simulink subsystem "PvtSubSys_LATC"  (R2020b)
settings: Solver=VariableStepAuto  StartTime=0.0  StopTime=10.0  RelTol=1e-3
undefined symbols (not defined in the file or in its folder): LCS_PLAN_PreViewIdxNum, LCS_PLAN_PreViewIdxSW_b, P_Global_CharSpd_ms, P_Global_SteeringAngleRatio, P_Global_WheelBase_m, P_LCS_DetNoOverRide_DrvTrq_TH, P_LCS_DetOverRide_DrvTrq_TH, P_LCS_ESS_AngleSlope_Limit, P_LCS_ESS_LogicTest_Enable, P_LCS_ESS_NotActiveFlgDelayTime, P_LCS_ESS_NotActiveFlgDelayTimeSW, P_LCS_ESS_SteerAngleErr, P_LCS_ESS_SteerAngleFilterTime, P_LCS_ESS_TarAngleFilterTime, P_LCS_ESSAngleSW, P_LCS_ESSOverrideTime1, P_LCS_ESSOverrideTime2, P_LCS_ESSOverrideTime3, P_LCS_ESSOverrideValue1, P_LCS_ESSOverrideValue2, P_LCS_IN_Offset_Test_SW, P_LCS_IN_Offset_Test_Value, P_LCS_LATC_AngleFilterTime_s, P_LCS_LATC_CurOffsetCurve_TabX_m, P_LCS_LATC_CurOffsetCurveFliterTime_Tab_s, P_LCS_LATC_CurOffsetVehicleSpdLimitValue_degs, P_LCS_LATC_DeltaEps_Tab_s, P_LCS_LATC_DxOffset_Sw, P_LCS_LATC_ELKAngleSlope_ratio, P_LCS_LATC_ELKMaxLatAcc_ms2, P_LCS_LATC_ESSA0Dis_TabX_m, P_LCS_LATC_ESSAddAngleSlope_Tab_degs, P_LCS_LATC_ESSAESAngleSlope_Tab_degs, P_LCS_LATC_ESSAngleSlope_ratio, P_LCS_LATC_ESSMaxLatAcc_ms2, P_LCS_LATC_LCAngleSlope_ratio, P_LCS_LATC_LCAngleSlope_Tab_degs, P_LCS_LATC_LCCancleMaxLatAcc_ms2, P_LCS_LATC_LCEcoAngleSlope_ratio, P_LCS_LATC_LCEcoAngleSlope_Tab_degs, P_LCS_LATC_LCEcoMaxLatAcc_ms2, P_LCS_LATC_LCKAngleSlope_ratio, P_LCS_LATC_LCKAngleSlope_Tab_degs, P_LCS_LATC_LCKIEAngleSlope_ratio, P_LCS_LATC_LCKIEAngleSlope_Tab_degs, P_LCS_LATC_LCKIEMaxLatAcc_ms2, P_LCS_LATC_LCKMaxLatAcc_ms2, P_LCS_LATC_LCNormalAngleSlope_ratio, P_LCS_LATC_LCNormalAngleSlope_Tab_degs, P_LCS_LATC_LCNormalMaxLatAcc_ms2, P_LCS_LATC_LCSportAngleSlope_ratio, P_LCS_LATC_LCSportAngleSlope_Tab_degs, P_LCS_LATC_LCSportMaxLatAcc_ms2, P_LCS_LATC_LKAAngleSlope_ratio, P_LCS_LATC_LKAAngleSlope_Tab_degs, P_LCS_LATC_LKAMaxLatAcc_ms2, P_LCS_LATC_MatrixQ1_st, P_LCS_LATC_MatrixQ3_st, P_LCS_LATC_MatrixR_st, P_LCS_LATC_MPCDeltaT_s ... (+70)
libraries: simulink x34
(part 1 of 5)
settings Model: Creator=GW00184765  LastModifiedBy=GW00201118

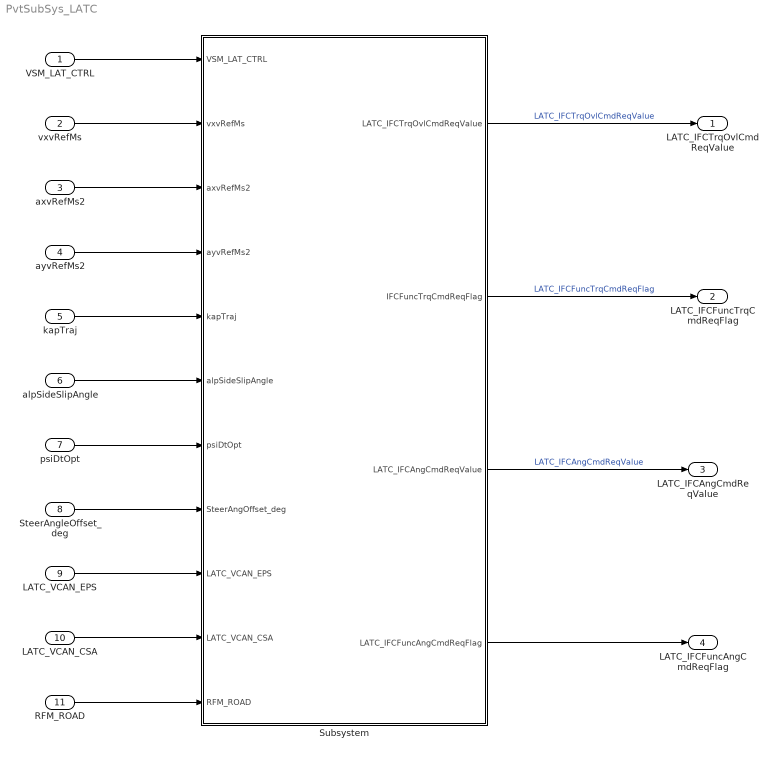
== system PvtSubSys_LATC ==
  VSM_LAT_CTRL : Inport  OutDataTypeStr=Bus: VSM_LAT_CTRL_BUS  PortDimensions=1  BusOutputAsStruct=on
  vxvRefMs : Inport  Port=2  OutDataTypeStr=single  PortDimensions=1  BusOutputAsStruct=on
  axvRefMs2 : Inport  Port=3  OutDataTypeStr=single  PortDimensions=1  BusOutputAsStruct=on
  ayvRefMs2 : Inport  Port=4  OutDataTypeStr=single  PortDimensions=1  BusOutputAsStruct=on
  kapTraj : Inport  Port=5  OutDataTypeStr=single  PortDimensions=1  BusOutputAsStruct=on
  alpSideSlipAngle : Inport  Port=6  OutDataTypeStr=single  PortDimensions=1  BusOutputAsStruct=on
  psiDtOpt : Inport  Port=7  OutDataTypeStr=single  PortDimensions=1  BusOutputAsStruct=on
  SteerAngleOffset_deg : Inport  Port=8  OutDataTypeStr=single  PortDimensions=1  BusOutputAsStruct=on
  LATC_VCAN_EPS : Inport  Port=9  OutDataTypeStr=Bus: VCAN_EPS_MSG_BUS  PortDimensions=1  BusOutputAsStruct=on
  LATC_VCAN_CSA : Inport  Port=10  OutDataTypeStr=Bus: VCAN_CSA_MSG_BUS  PortDimensions=1  BusOutputAsStruct=on
  RFM_ROAD : Inport  Port=11  OutDataTypeStr=Bus: RFM_ROAD_BUS  PortDimensions=1  BusOutputAsStruct=on
  Subsystem : Subsystem
  LATC_IFCTrqOvlCmdReqValue : Outport  OutDataTypeStr=single  PortDimensions=1  BusOutputAsStruct=on
  LATC_IFCFuncTrqCmdReqFlag : Outport  Port=2  OutDataTypeStr=uint8  PortDimensions=1  BusOutputAsStruct=on
  LATC_IFCAngCmdReqValue : Outport  Port=3  OutDataTypeStr=single  PortDimensions=1  BusOutputAsStruct=on
  LATC_IFCFuncAngCmdReqFlag : Outport  Port=4  OutDataTypeStr=uint8  PortDimensions=1  BusOutputAsStruct=on
  wires:
  Subsystem/1(LATC_IFCTrqOvlCmdReqValue) -> LATC_IFCTrqOvlCmdReqValue/1  "LATC_IFCTrqOvlCmdReqValue"
  RFM_ROAD/1 -> Subsystem/11(RFM_ROAD)
  kapTraj/1 -> Subsystem/5(kapTraj)
  vxvRefMs/1 -> Subsystem/2(vxvRefMs)
  alpSideSlipAngle/1 -> Subsystem/6(alpSideSlipAngle)
  ayvRefMs2/1 -> Subsystem/4(ayvRefMs2)
  LATC_VCAN_EPS/1 -> Subsystem/9(LATC_VCAN_EPS)
  Subsystem/2(IFCFuncTrqCmdReqFlag) -> LATC_IFCFuncTrqCmdReqFlag/1  "LATC_IFCFuncTrqCmdReqFlag"
  psiDtOpt/1 -> Subsystem/7(psiDtOpt)
  SteerAngleOffset_deg/1 -> Subsystem/8(SteerAngOffset_deg)
  VSM_LAT_CTRL/1 -> Subsystem/1(VSM_LAT_CTRL)
  axvRefMs2/1 -> Subsystem/3(axvRefMs2)
  LATC_VCAN_CSA/1 -> Subsystem/10(LATC_VCAN_CSA)
  Subsystem/3(LATC_IFCAngCmdReqValue) -> LATC_IFCAngCmdReqValue/1  "LATC_IFCAngCmdReqValue"
  Subsystem/4(LATC_IFCFuncAngCmdReqFlag) -> LATC_IFCFuncAngCmdReqFlag/1

== system PvtSubSys_LATC/Subsystem ==
  VSM_LAT_CTRL : Inport  OutDataTypeStr=Bus: VSM_LAT_CTRL_BUS  PortDimensions=1  Interpolate=off  BusOutputAsStruct=on
  vxvRefMs : Inport  Port=2  OutDataTypeStr=single  PortDimensions=1  Interpolate=off  BusOutputAsStruct=on
  axvRefMs2 : Inport  Port=3  OutDataTypeStr=single  PortDimensions=1  Interpolate=off  BusOutputAsStruct=on
  ayvRefMs2 : Inport  Port=4  OutDataTypeStr=single  PortDimensions=1  Interpolate=off  BusOutputAsStruct=on
  kapTraj : Inport  Port=5  OutDataTypeStr=single  PortDimensions=1  Interpolate=off  BusOutputAsStruct=on
  alpSideSlipAngle : Inport  Port=6  OutDataTypeStr=single  PortDimensions=1  Interpolate=off  BusOutputAsStruct=on
  psiDtOpt : Inport  Port=7  OutDataTypeStr=single  PortDimensions=1  Interpolate=off  BusOutputAsStruct=on
  SteerAngOffset_deg : Inport  Port=8  OutDataTypeStr=single  PortDimensions=1  Interpolate=off  BusOutputAsStruct=on
  LATC_VCAN_EPS : Inport  Port=9  OutDataTypeStr=Bus: VCAN_EPS_MSG_BUS  PortDimensions=1  BusOutputAsStruct=on
  LATC_VCAN_CSA : Inport  Port=10  OutDataTypeStr=Bus: VCAN_CSA_MSG_BUS  PortDimensions=1  BusOutputAsStruct=on
  RFM_ROAD : Inport  Port=11  OutDataTypeStr=Bus: RFM_ROAD_BUS  PortDimensions=1  BusOutputAsStruct=on
  Bus Creator : BusCreator  Inputs=8
  Constant : Constant  Value=0  OutDataTypeStr=single
  Constant1 : Constant  Value=0  OutDataTypeStr=boolean
  Constant2 : Constant  Value=0  OutDataTypeStr=single
  Constant3 : Constant  Value=0  OutDataTypeStr=uint8
  Constant4 : Constant  Value=0  OutDataTypeStr=single
  Constant5 : Constant  Value=0  OutDataTypeStr=uint8
  Constant8 : Constant  Value=P_LCS_Trq_Switch  OutDataTypeStr=uint8
  Counter Limited : simulink/Sources/Counter Limited  uplimit=15  tsamp=-1
  LateralControl : Subsystem
  SW_Branch : Constant  Value=303  OutDataTypeStr=uint32
  SW_VERSION : Constant  Value=38300517  OutDataTypeStr=uint32
  Switch{1..4} (4 alike) : Switch  Criteria=u2 ~= 0
  Terminator{,1..3} (4 alike) : Terminator
  LATC_IFCTrqOvlCmdReqValue : Outport  OutDataTypeStr=single  PortDimensions=1  BusOutputAsStruct=on
  IFCFuncTrqCmdReqFlag : Outport  Port=2  OutDataTypeStr=uint8  PortDimensions=1  BusOutputAsStruct=on
  LATC_IFCAngCmdReqValue : Outport  Port=3  OutDataTypeStr=single  PortDimensions=1  BusOutputAsStruct=on
  LATC_IFCFuncAngCmdReqFlag : Outport  Port=4  OutDataTypeStr=uint8  PortDimensions=1  BusOutputAsStruct=on
  wires:
  Counter Limited/1 -> Terminator/1  "LCS_Counter"
  LATC_VCAN_CSA/1 -> LateralControl/10(LATC_VCAN_CSA)
  VSM_LAT_CTRL/1 -> LateralControl/1(VSM_LAT_CTRL)
  psiDtOpt/1 -> LateralControl/7(psiDtOpt)
  ayvRefMs2/1 -> LateralControl/4(ayvRefMs2)
  RFM_ROAD/1 -> LateralControl/11(RFM_ROAD)
  SteerAngOffset_deg/1 -> LateralControl/8(SteerAngOffset_deg)
  vxvRefMs/1 -> LateralControl/2(vxvRefMs)
  kapTraj/1 -> LateralControl/5(kapTraj)
  alpSideSlipAngle/1 -> LateralControl/6(alpSideSlipAngle)
  axvRefMs2/1 -> LateralControl/3(axvRefMs2)
  LATC_VCAN_EPS/1 -> LateralControl/9(LATC_VCAN_EPS)
  Constant2/1 -> Bus Creator/1  "HWP_AngCmdReqVal"
  LateralControl/5(HWP_ReqCtrlEPS) -> Bus Creator/3  "HWP_ReqCtrlEPS"
  LateralControl/6(HWP_ReqCtrlEPSVld) -> Bus Creator/4  "HWP_ReqCtrlEPSVld"
  LateralControl/7(HWP_WorkReq) -> Bus Creator/5  "HWP_WorkReq"
  LateralControl/8(HWP_WorkReqVld) -> Bus Creator/6  "HWP_WorkReqVld"
  Constant3/1 -> Bus Creator/7  "HWP_FuncTrqCmdReqFlag"
  Constant4/1 -> Bus Creator/8  "HWP_TrqOvlCmdReqValue"
  Constant1/1 -> Bus Creator/2  "HWP_AngCmdReqValVld"
  SW_VERSION/1 -> Terminator1/1  "LCS_SubModel_VERSION"
  SW_Branch/1 -> Terminator2/1  "LCS_SubModel_Number"
  LateralControl/1(TrqCmdReqVal) -> Switch2/1
  LateralControl/2(TrqCmdReqValVld) -> Switch3/1
  Constant/1 -> Switch2/3, Switch1/1
  Constant5/1 -> Switch4/1, Switch3/3
  Constant8/1 -> Switch3/2, Switch4/2, Switch1/2, Switch2/2  "LCS_Trq_Switch"
  Switch2/1 -> LATC_IFCTrqOvlCmdReqValue/1
  Switch1/1 -> LATC_IFCAngCmdReqValue/1
  LateralControl/3(AngCmdReqVal) -> Switch1/3  "HWP_AngCmdReqVal"
  Switch3/1 -> IFCFuncTrqCmdReqFlag/1
  Switch4/1 -> LATC_IFCFuncAngCmdReqFlag/1
  LateralControl/4(AngCmdReqValVld) -> Switch4/3  "HWP_AngCmdReqValVld"
  Bus Creator/1 -> Terminator3/1

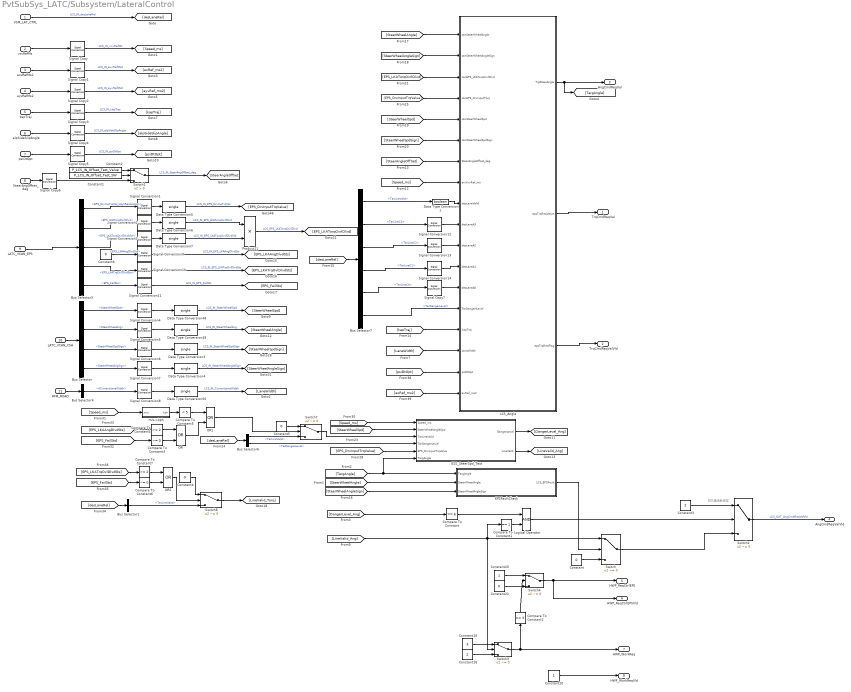
== system PvtSubSys_LATC/Subsystem/LateralControl ==
  note: ESS激活标志位
  VSM_LAT_CTRL : Inport  OutDataTypeStr=Bus: VSM_LAT_CTRL_BUS  PortDimensions=1  BusOutputAsStruct=on
  vxvRefMs : Inport  Port=2  OutDataTypeStr=single  PortDimensions=1  BusOutputAsStruct=on
  axvRefMs2 : Inport  Port=3  OutDataTypeStr=single  PortDimensions=1  BusOutputAsStruct=on
  ayvRefMs2 : Inport  Port=4  OutDataTypeStr=single  PortDimensions=1  BusOutputAsStruct=on
  kapTraj : Inport  Port=5  OutDataTypeStr=single  PortDimensions=1  BusOutputAsStruct=on
  alpSideSlipAngle : Inport  Port=6  OutDataTypeStr=single  PortDimensions=1  BusOutputAsStruct=on
  psiDtOpt : Inport  Port=7  OutDataTypeStr=single  PortDimensions=1  BusOutputAsStruct=on
  SteerAngOffset_deg : Inport  Port=8  OutDataTypeStr=single  PortDimensions=1  BusOutputAsStruct=on
  LATC_VCAN_EPS : Inport  Port=9  OutDataTypeStr=Bus: VCAN_EPS_MSG_BUS  PortDimensions=1  BusOutputAsStruct=on
  LATC_VCAN_CSA : Inport  Port=10  OutDataTypeStr=Bus: VCAN_CSA_MSG_BUS  PortDimensions=1  BusOutputAsStruct=on
  RFM_ROAD : Inport  Port=11  OutDataTypeStr=Bus: RFM_ROAD_BUS  PortDimensions=1  BusOutputAsStruct=on
  Bus Selector : BusSelector  OutputSignals=SteerWheelSpd,SteerWheelAng,SteerWheelSpdSign,SteerWheelAngSign
  Bus Selector1 : BusSelector  OutputSignals=TarLineValid
  Bus Selector3 : BusSelector  OutputSignals=EPS_DrvInpTrqVal_HighReslolution,EPS_LKATorqOvrlDlvd,EPS_LKATorqOvrlDlvdVld,EPS_LKATrqOvlDlvdSts,EPS_FailSts
  Bus Selector4 : BusSelector  OutputSignals=dCurrentLaneWidth
  Bus Selector6 : BusSelector  OutputSignals=TarLineValid,TarDangerLevel
  Bus Selector7 : BusSelector  OutputSignals=TarLineValid,TarLineC3,TarLineC2,TarLineC1,TarLineC0,TarDangerLevel
  Compare To Constant : simulink/Logic and Bit Operations/Compare To Constant  relop===  const=6  OutDataTypeStr=boolean
  Compare To Constant1 : simulink/Logic and Bit Operations/Compare To Constant  relop===  const=1  OutDataTypeStr=boolean
  Compare To Constant2 : simulink/Logic and Bit Operations/Compare To Constant  relop===  const=3  OutDataTypeStr=boolean
  Compare To Constant3 : simulink/Logic and Bit Operations/Compare To Constant  relop=~=  const=0  OutDataTypeStr=boolean
  Compare To Constant4 : simulink/Logic and Bit Operations/Compare To Constant  relop=>=  const=2  OutDataTypeStr=boolean
  Compare To Constant5 : simulink/Logic and Bit Operations/Compare To Constant  relop=<  const=5  OutDataTypeStr=boolean
  Compare To Constant6 : simulink/Logic and Bit Operations/Compare To Constant  relop=~=  const=0  OutDataTypeStr=boolean
  Compare To Constant7 : simulink/Logic and Bit Operations/Compare To Constant  relop=>=  const=2  OutDataTypeStr=boolean
  Constant : Constant  Value=0  OutDataTypeStr=uint8
  Constant1 : Constant  Value=P_LCS_IN_Offset_Test_SW  OutDataTypeStr=uint8
  Constant10 : Constant  OutDataTypeStr=boolean
  Constant15 : Constant  Value=3  OutDataTypeStr=uint8
  Constant16 : Constant  Value=2  OutDataTypeStr=uint8
  Constant2 : Constant  Value=P_LCS_IN_Offset_Test_Value  OutDataTypeStr=single
  Constant20 : Constant  OutDataTypeStr=boolean
  Constant21 : Constant  Value=0  OutDataTypeStr=boolean
  Constant3 : Constant  Value=2  OutDataTypeStr=uint8
  Constant4 : Constant  Value=0  OutDataTypeStr=boolean
  Constant5 : Constant  Value=0  OutDataTypeStr=boolean
  Constant6 : Constant  Value=0  OutDataTypeStr=uint8
  Data Type Conversion1 : DataTypeConversion  OutDataTypeStr=boolean
  Data Type Conversion{3..7,48..50} (8 alike) : DataTypeConversion  OutDataTypeStr=single
  EPSFaultCheck : Subsystem
  ESS_SteerSpd_Test : Subsystem
  LCS_Angle : Subsystem
  Logical Operator : Logic  AllPortsSameDT=off  OutDataTypeStr=boolean
  OR : Logic  Operator=OR  AllPortsSameDT=off  OutDataTypeStr=boolean
  OR1 : Logic  Operator=OR  AllPortsSameDT=off  OutDataTypeStr=boolean
  OR2 : Logic  Operator=OR  AllPortsSameDT=off  OutDataTypeStr=boolean
  Product11 : Product
  Signal Conversion{1..14} (14 alike) : SignalConversion  OverrideOpt=off
  Signal Copy{,1..7} (8 alike) : SignalConversion  OverrideOpt=off
  Switch{,2..4} (4 alike) : Switch  Criteria=u2 ~= 0
  Switch1 : Switch  Criteria=u2 > Threshold
  Switch7 : Switch  Criteria=u2 ~= 0  Threshold=5
  Switch8 : Switch  Criteria=u2 ~= 0  Threshold=5
  m/s->kph : Subsystem
  TrqCmdReqVal : Outport  OutDataTypeStr=single
  TrqCmdReqValVld : Outport  Port=2  OutDataTypeStr=uint8
  AngCmdReqVal : Outport  Port=3  OutDataTypeStr=single
  AngCmdReqValVld : Outport  Port=4
  HWP_ReqCtrlEPS : Outport  Port=5
  HWP_ReqCtrlEPSVld : Outport  Port=6
  HWP_WorkReq : Outport  Port=7
  HWP_WorkReqVld : Outport  Port=8
  wires:
  Signal Copy7/1 -> LCS_Angle/13(desLaneA0)
  Signal Conversion14/1 -> LCS_Angle/12(desLaneA1)
  Signal Conversion13/1 -> LCS_Angle/11(desLaneA2)
  Signal Conversion12/1 -> LCS_Angle/10(desLaneA3)
  [axRef_ms2] -> LCS_Angle/18(axRef_ms2)
  [psiDtOpt] -> LCS_Angle/17(psiDtOpt)
  Switch8/1 -> [LineValid_Torq]
  Constant4/1 -> Switch8/1
  OR2/1 -> Switch8/2
  [EPS_FailSts] -> Compare To Constant6/1
  [EPS_LKATrqOvlDlvdSts] -> Compare To Constant7/1
  Compare To Constant6/1 -> OR2/2
  Compare To Constant7/1 -> OR2/1
  [desLaneRel] -> Bus Selector1/1
  Bus Selector1/1 -> Switch8/3  "<TarLineValid>"
  OR1/1 -> Switch7/2
  OR/1 -> OR1/2
  Compare To Constant5/1 -> OR1/1
  Compare To Constant4/1 -> OR/1
  Compare To Constant3/1 -> OR/2
  [EPS_LKAAngDlvdSts] -> Compare To Constant4/1
  [EPS_FailSts] -> Compare To Constant3/1
  Signal Conversion11/1 -> [EPS_FailSts]  "LCS_IN_EPS_FailSts"
  Signal Conversion10/1 -> [EPS_LKATrqOvlDlvdSts]  "LCS_IN_EPS_LKATrqOvlDlvdSts"
  Signal Conversion9/1 -> [EPS_LKAAngDlvdSts]  "LCS_IN_EPS_LKAAngDlvdSts"
  Bus Selector3/5 -> Signal Conversion11/1  "<EPS_FailSts>"
  Bus Selector3/4 -> Signal Conversion10/1  "<EPS_LKATrqOvlDlvdSts>"
  Constant6/1 -> Signal Conversion9/1  "<EPS_LKAAngDlvdSts>"
  Switch7/1 -> ESS_SteerSpd_Test/3(TarLineValid)
  m/s->kph/1(kph) -> Compare To Constant5/1
  [Speed_ms] -> m/s->kph/1(m/s)
  Constant5/1 -> Switch7/1
  Bus Selector6/1 -> Switch7/3  "<TarLineValid>"
  [Speed_ms] -> ESS_SteerSpd_Test/1(Speed_ms)
  [EPS_DrvInputTrqValue] -> ESS_SteerSpd_Test/5(EPS_DrvInputTrqValue)
  Bus Selector7/6 -> LCS_Angle/14(TarDangerlLevel)  "<TarDangerLevel>"
  [TargAngle] -> EPSFaultCheck/1(TargAngle), ESS_SteerSpd_Test/6(TargAngle)
  [SteerWheelSpd] -> ESS_SteerSpd_Test/2(SteerWheelAngleSpd)
  [desLaneRel] -> Bus Selector6/1
  Bus Selector6/2 -> ESS_SteerSpd_Test/4(TarDangerLevel)  "<TarDangerLevel>"
  ESS_SteerSpd_Test/1(DangerLevel) -> [DangerLevel_Ang]
  ESS_SteerSpd_Test/2(LineValid) -> [LineValid_Ang]
  Constant3/1 -> Switch2/1
  Switch/1 -> Switch2/3
  Logical Operator/1 -> Switch2/2
  Compare To Constant1/1 -> Logical Operator/2
  Compare To Constant/1 -> Logical Operator/1
  [DangerLevel_Ang] -> Compare To Constant/1
  Signal Conversion8/1 -> Data Type Conversion50/1
  Signal Conversion7/1 -> Data Type Conversion4/1
  Signal Conversion6/1 -> Data Type Conversion3/1
  Signal Conversion5/1 -> Data Type Conversion49/1
  Signal Conversion4/1 -> Data Type Conversion48/1
  Signal Conversion3/1 -> Data Type Conversion7/1
  Signal Conversion2/1 -> Data Type Conversion6/1
  Signal Conversion1/1 -> Data Type Conversion5/1
  Constant2/1 -> Switch1/1
  Constant1/1 -> Switch1/2
  Signal Copy6/1 -> Switch1/3
  [LaneWidth] -> LCS_Angle/16(LaneWidth)
  Switch1/1 -> [SteerAngleOffSet]  "LCS_IN_SteerAngOffset_deg"
  Signal Copy5/1 -> [psiDtOpt]  "LCS_IN_psiDtOpt"
  Signal Copy4/1 -> [alpSideSlipAngle]  "LCS_IN_alpSideSlipAngle"
  Signal Copy3/1 -> [kapTraj]  "LCS_IN_kapTraj"
  Signal Copy2/1 -> [ayvRef_ms2]  "LCS_IN_ayvRefMs2"
  Signal Copy1/1 -> [axRef_ms2]  "LCS_IN_axvRefMs2"
  Signal Copy/1 -> [Speed_ms]  "LCS_IN_vxvRefMs"
  LATC_VCAN_CSA/1 -> Bus Selector/1
  LATC_VCAN_EPS/1 -> Bus Selector3/1
  Product11/1 -> [EPS_LKATorqOvrlDlvd]  "LCS_EPS_LKATorqOvrlDlvd"
  Data Type Conversion50/1 -> [LaneWidth]  "LCS_IN_CurrentLaneWidth"
  Data Type Conversion49/1 -> [SteerWheelAngle]  "LCS_IN_SteerWheelAng"
  Data Type Conversion48/1 -> [SteerWheelSpd]  "LCS_IN_SteerWheelSpd"
  psiDtOpt/1 -> Signal Copy5/1
  alpSideSlipAngle/1 -> Signal Copy4/1
  kapTraj/1 -> Signal Copy3/1
  ayvRefMs2/1 -> Signal Copy2/1
  Bus Selector4/1 -> Signal Conversion8/1  "<dCurrentLaneWidth>"
  RFM_ROAD/1 -> Bus Selector4/1
  Bus Selector3/3 -> Signal Conversion3/1  "<EPS_LKATorqOvrlDlvdVld>"
  Bus Selector3/2 -> Signal Conversion2/1  "<EPS_LKATorqOvrlDlvd>"
  Bus Selector3/1 -> Signal Conversion1/1  "<EPS_DrvInpTrqVal_HighReslolution>"
  Bus Selector/4 -> Signal Conversion7/1  "<SteerWheelAngSign>"
  Bus Selector/3 -> Signal Conversion6/1  "<SteerWheelSpdSign>"
  Bus Selector/1 -> Signal Conversion4/1  "<SteerWheelSpd>"
  Bus Selector/2 -> Signal Conversion5/1  "<SteerWheelAng>"
  SteerAngOffset_deg/1 -> Signal Copy6/1
  axvRefMs2/1 -> Signal Copy1/1
  vxvRefMs/1 -> Signal Copy/1
  Data Type Conversion7/1 -> Product11/2  "LCS_IN_EPS_LKATorqOvrlDlvdVld"
  Data Type Conversion6/1 -> Product11/1  "LCS_IN_EPS_LKATorqOvrlDlvd"
  Data Type Conversion5/1 -> [EPS_DrvInputTrqValue]  "LCS_IN_EPS_DrvInpTrqVal"
  Data Type Conversion4/1 -> [SteerWheelAngleSign]  "LCS_IN_SteerWheelAngleSign"
  Data Type Conversion3/1 -> [SteerWheelSpdSign]  "LCS_IN_SteerWheelSpdSign"
  VSM_LAT_CTRL/1 -> [desLaneRel]  "LCS_IN_desLaneRel"
  Bus Selector7/3 -> Signal Conversion13/1  "<TarLineC2>"
  LCS_Angle/1(TrgSteerAngle) -> [TargAngle], AngCmdReqVal/1
  [kapTraj] -> LCS_Angle/15(kapTraj)
  [EPS_DrvInputTrqValue] -> LCS_Angle/4(canEPS_DrvInputTorq)
  [EPS_LKATorqOvrlDlvd] -> LCS_Angle/3(canEPS_LKATorqOvrlDlvd)
  Bus Selector7/2 -> Signal Conversion12/1  "<TarLineC3>"
  [desLaneRel] -> Bus Selector7/1
  [LineValid_Ang] -> Switch3/2, Switch/1, Compare To Constant1/1
  [SteerAngleOffSet] -> LCS_Angle/7(SteerAngleOffset_deg)
  Bus Selector7/4 -> Signal Conversion14/1  "<TarLineC1>"
  Bus Selector7/5 -> Signal Copy7/1  "<TarLineC0>"
  [SteerWheelSpdSign] -> LCS_Angle/6(canSteerWheelSpdSign)
  [SteerWheelAngleSign] -> LCS_Angle/2(canSteerWheelAngleSign)
  [Speed_ms] -> LCS_Angle/8(eviVxvRef_ms)
  [SteerWheelSpd] -> LCS_Angle/5(canSteerWheelSpd)
  [SteerWheelAngle] -> LCS_Angle/1(canSteerWheelAngle)
  Bus Selector7/1 -> Data Type Conversion1/1  "<TarLineValid>"
  Constant10/1 -> HWP_WorkReqVld/1
  Constant16/1 -> Switch3/3
  Switch4/1 -> HWP_ReqCtrlEPSVld/1, HWP_ReqCtrlEPS/1
  Constant15/1 -> Switch3/1
  Compare To Constant2/1 -> Switch4/2
  Constant20/1 -> Switch4/1
  Constant21/1 -> Switch4/3
  Switch3/1 -> HWP_WorkReq/1, Compare To Constant2/1
  Switch2/1 -> AngCmdReqValVld/1  "LCS_OUT_AngCmdReqValVld"
  Constant/1 -> Switch/3
  [SteerWheelAngle] -> EPSFaultCheck/2(SteerWheelAngle)
  [SteerWheelAngleSign] -> EPSFaultCheck/3(SteerWheelAngleSign)
  EPSFaultCheck/1(LCS_EPSFault) -> Switch/2
  Data Type Conversion1/1 -> LCS_Angle/9(desLaneValid)
  LCS_Angle/3(epsTrqReqFlag) -> TrqCmdReqValVld/1
  LCS_Angle/2(epsTrqReqValue) -> TrqCmdReqVal/1

== system PvtSubSys_LATC/Subsystem/LateralControl/EPSFaultCheck ==
  TargAngle : Inport
  SteerWheelAngle : Inport  Port=2
  SteerWheelAngleSign : Inport  Port=3
  Abs : Abs
  Add2 : Sum  Inputs=+-
  Add3 : Sum  Inputs=+-
  Compare To Constant3 : simulink/Logic and Bit Operations/Compare To Constant  relop=>=  const=15  OutDataTypeStr=boolean
  Constant24 : Constant  Value=0.5
  Gain1 : Gain  Gain=-2
  Logical Operator2 : Logic  Inputs=3  AllPortsSameDT=off  OutDataTypeStr=boolean
  MATLAB Function1 : MATLAB Function  TreatAsAtomicUnit=on
  Product1 : Product
  Unit Delay1 : UnitDelay  SampleTime=-1  HasFrameUpgradeWarning=on
  Unit Delay2 : UnitDelay  SampleTime=-1  HasFrameUpgradeWarning=on
  Unit Delay4 : UnitDelay  InitialCondition=1  SampleTime=-1  HasFrameUpgradeWarning=on
  LCS_EPSFault : Outport
  wires:
  Abs/1 -> Compare To Constant3/1
  Unit Delay1/1 -> Unit Delay2/1, Logical Operator2/2
  MATLAB Function1/2(count) -> Unit Delay4/1
  Product1/1 -> Add2/2
  Unit Delay2/1 -> Logical Operator2/3
  Compare To Constant3/1 -> Unit Delay1/1, Logical Operator2/1
  TargAngle/1 -> Add2/1
  Add2/1 -> Abs/1
  Gain1/1 -> Product1/2
  Constant24/1 -> Add3/2
  Add3/1 -> Gain1/1
  Logical Operator2/1 -> MATLAB Function1/1(u)
  Unit Delay4/1 -> MATLAB Function1/2(countK)
  SteerWheelAngle/1 -> Product1/1
  SteerWheelAngleSign/1 -> Add3/1
  MATLAB Function1/1(y) -> LCS_EPSFault/1  "LCS_EPSFault"

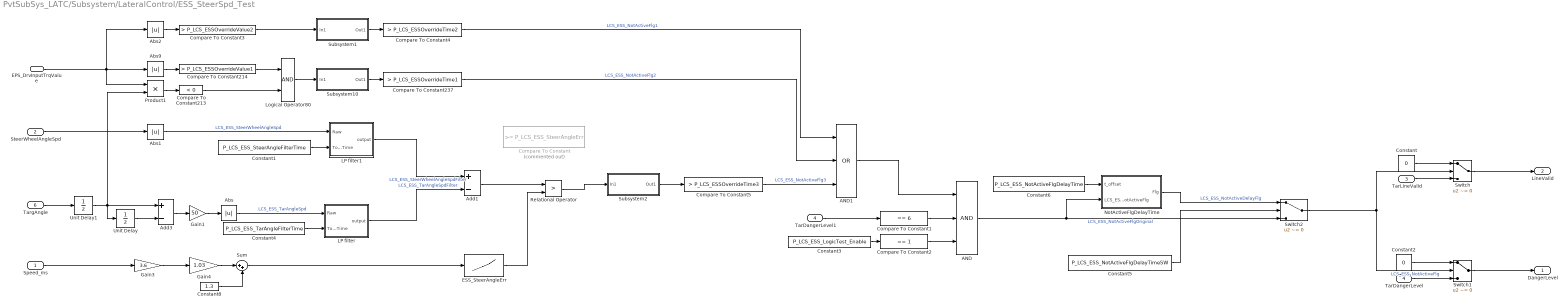
== system PvtSubSys_LATC/Subsystem/LateralControl/ESS_SteerSpd_Test ==
  Speed_ms : Inport
  SteerWheelAngleSpd : Inport  Port=2
  TarLineValid : Inport  Port=3
  TarDangerLevel : Inport  Port=4
  EPS_DrvInputTrqValue : Inport  Port=5
  TargAngle : Inport  Port=6
  AND : Logic  Inputs=3  AllPortsSameDT=off  OutDataTypeStr=boolean
  AND1 : Logic  Operator=OR  Inputs=3  AllPortsSameDT=off  OutDataTypeStr=boolean
  Abs{,1..2,9} (4 alike) : Abs
  Add1 : Sum  Inputs=+-
  Add3 : Sum  Inputs=+-
  Compare To Constant : simulink/Logic and Bit Operations/Compare To Constant  Commented=on  relop=>=  const=P_LCS_ESS_SteerAngleErr  OutDataTypeStr=boolean
  Compare To Constant1 : simulink/Logic and Bit Operations/Compare To Constant  relop===  const=6  OutDataTypeStr=boolean
  Compare To Constant2 : simulink/Logic and Bit Operations/Compare To Constant  relop===  const=1  OutDataTypeStr=boolean
  Compare To Constant213 : simulink/Logic and Bit Operations/Compare To Constant  relop=<  const=0  OutDataTypeStr=boolean
  Compare To Constant214 : simulink/Logic and Bit Operations/Compare To Constant  relop=>  const=P_LCS_ESSOverrideValue1  OutDataTypeStr=boolean
  Compare To Constant237 : simulink/Logic and Bit Operations/Compare To Constant  relop=>  const=P_LCS_ESSOverrideTime1  OutDataTypeStr=boolean
  Compare To Constant3 : simulink/Logic and Bit Operations/Compare To Constant  relop=>  const=P_LCS_ESSOverrideValue2  OutDataTypeStr=boolean
  Compare To Constant4 : simulink/Logic and Bit Operations/Compare To Constant  relop=>  const=P_LCS_ESSOverrideTime2  OutDataTypeStr=boolean
  Compare To Constant5 : simulink/Logic and Bit Operations/Compare To Constant  relop=>  const=P_LCS_ESSOverrideTime3  OutDataTypeStr=boolean
  Constant : Constant  Value=0  OutDataTypeStr=boolean
  Constant1 : Constant  Value=P_LCS_ESS_SteerAngleFilterTime  OutDataTypeStr=single
  Constant2 : Constant  Value=0  OutDataTypeStr=uint8
  Constant3 : Constant  Value=P_LCS_ESS_LogicTest_Enable  OutDataTypeStr=boolean
  Constant4 : Constant  Value=P_LCS_ESS_TarAngleFilterTime  OutDataTypeStr=single
  Constant5 : Constant  Value=P_LCS_ESS_NotActiveFlgDelayTimeSW  OutDataTypeStr=single
  Constant6 : Constant  Value=P_LCS_ESS_NotActiveFlgDelayTime  OutDataTypeStr=single
  Constant8 : Constant  Value=1.3  OutDataTypeStr=single
  ESS_SteerAngleErr : Lookup_n-D  NumberOfTableDimensions=1  BreakpointsForDimension1=P_LCS_LATC_VehicleSpd_TabX_Kph  Table=P_LCS_ESS_SteerAngleErr  ExtrapMethod=Clip  InternalRulePriority=Speed  RndMeth=Simplest  InputSameDT=on
  Gain1 : Gain  Gain=50
  Gain3 : Gain  Gain=3.6
  Gain4 : Gain  Gain=1.03
  LP filter : Subsystem
  LP filter1 : Subsystem
  Logical Operator80 : Logic  AllPortsSameDT=off  OutDataTypeStr=boolean
  NotActiveFlgDelayTime : Subsystem
  Product1 : Product
  Relational Operator : RelationalOperator  Operator=>  OutDataTypeStr=boolean  RndMeth=Simplest
  Subsystem1 : Subsystem  mask{Ts=0.02, Max=10}
      mask prompts: Ts "Sample Time:"; Max "Max Limit:"
      mask Display:
      | Ts=get_param(gcb,'Ts');
      | Max=get_param(gcb,'Max');
      | disp(['Ts:' Ts '\n' 'Max:' Max ]);
  Subsystem10 : Subsystem  mask{Ts=0.02, Max=10}
      mask prompts: Ts "Sample Time:"; Max "Max Limit:"
      mask Display:
      | Ts=get_param(gcb,'Ts');
      | Max=get_param(gcb,'Max');
      | disp(['Ts:' Ts '\n' 'Max:' Max ]);
  Subsystem2 : Subsystem  mask{Ts=0.02, Max=10}
      mask prompts: Ts "Sample Time:"; Max "Max Limit:"
      mask Display:
      | Ts=get_param(gcb,'Ts');
      | Max=get_param(gcb,'Max');
      | disp(['Ts:' Ts '\n' 'Max:' Max ]);
  Sum : Sum  Inputs=|++
  Switch : Switch  Criteria=u2 ~= 0
  Switch1 : Switch  Criteria=u2 ~= 0
  Switch2 : Switch  Criteria=u2 ~= 0
  TarDangerLevel1 : InportShadow  Port=4
  Unit Delay : UnitDelay  SampleTime=-1  HasFrameUpgradeWarning=on
  Unit Delay1 : UnitDelay  SampleTime=-1  HasFrameUpgradeWarning=on
  DangerLevel : Outport
  LineValid : Outport  Port=2
  wires:
  Subsystem2/1(Out1) -> Compare To Constant5/1
  Sum/1 -> ESS_SteerAngleErr/1
  Speed_ms/1 -> Gain3/1
  Constant8/1 -> Sum/2
  Gain4/1 -> Sum/1
  Gain3/1 -> Gain4/1
  ESS_SteerAngleErr/1 -> Relational Operator/2
  NotActiveFlgDelayTime/1(Flg) -> Switch2/1  "LCS_ESS_NotActiveDelayFlg"
  Constant5/1 -> Switch2/2
  AND/1 -> NotActiveFlgDelayTime/2(LCS_ESS_NotActiveFlg), Switch2/3  "LCS_ESS_NotActiveFlgOriginal"
  Constant6/1 -> NotActiveFlgDelayTime/1(t_offset)
  AND1/1 -> AND/1
  Compare To Constant5/1 -> AND1/3  "LCS_ESS_NotActiveFlg3"
  Compare To Constant4/1 -> AND1/1  "LCS_ESS_NotActiveFlg1"
  Subsystem1/1(Out1) -> Compare To Constant4/1
  Compare To Constant3/1 -> Subsystem1/1(In1)
  Abs2/1 -> Compare To Constant3/1
  TargAngle/1 -> Unit Delay1/1
  Compare To Constant237/1 -> AND1/2  "LCS_ESS_NotActiveFlg2"
  Subsystem10/1(Out1) -> Compare To Constant237/1
  Logical Operator80/1 -> Subsystem10/1(In1)
  EPS_DrvInputTrqValue/1 -> Product1/1, Abs9/1, Abs2/1
  Unit Delay1/1 -> Unit Delay/1, Product1/2, Add3/1
  Compare To Constant213/1 -> Logical Operator80/2
  Product1/1 -> Compare To Constant213/1
  Abs9/1 -> Compare To Constant214/1
  Compare To Constant214/1 -> Logical Operator80/1
  Abs/1 -> LP filter/1(Raw)  "LCS_ESS_TarAngleSpd"
  Add3/1 -> Gain1/1
  SteerWheelAngleSpd/1 -> Abs1/1
  Unit Delay/1 -> Add3/2
  Constant4/1 -> LP filter/2(TorqFilterTime)
  Constant1/1 -> LP filter1/2(TorqFilterTime)
  Gain1/1 -> Abs/1
  Abs1/1 -> LP filter1/1(Raw)  "LCS_ESS_SteerWheelAngleSpd"
  LP filter1/1(output) -> Add1/1  "LCS_ESS_SteerWheelAngleSpdFilter"
  LP filter/1(output) -> Add1/2  "LCS_ESS_TarAngleSpdFilter"
  Add1/1 -> Relational Operator/1
  Switch2/1 -> Switch/2, Switch1/2  "LCS_ESS_NotActiveFlg"
  Constant/1 -> Switch/1
  Constant2/1 -> Switch1/1
  Relational Operator/1 -> Subsystem2/1(In1)
  Compare To Constant1/1 -> AND/2
  Compare To Constant2/1 -> AND/3
  Constant3/1 -> Compare To Constant2/1
  TarLineValid/1 -> Switch/3
  TarDangerLevel/1 -> Switch1/3
  TarDangerLevel1/1 -> Compare To Constant1/1
  Switch/1 -> LineValid/1
  Switch1/1 -> DangerLevel/1

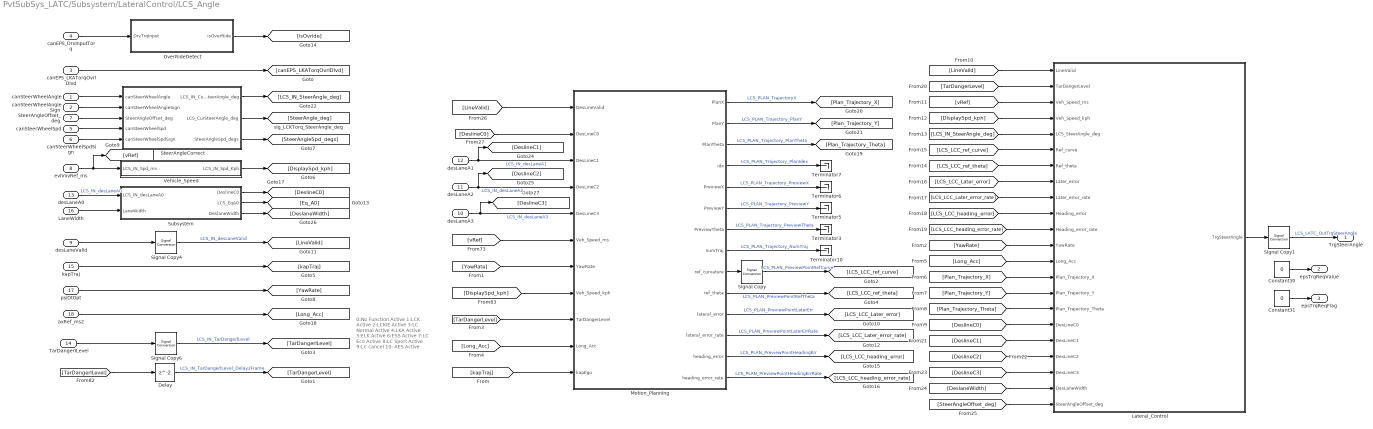
== system PvtSubSys_LATC/Subsystem/LateralControl/LCS_Angle ==
  note: 0:No Function Active
      | 1:LCK Active
      | 2:LCKIE Active
      | 3:LC Normal Active
      | 4:LKA Active
      | 5:ELK Active
      | 6:ESS Active
      | 7:LC Eco Active
      | 8:LC Sport Active
      | 9:LC cancel
      | 10: AES Active
  canSteerWheelAngle : Inport
  canSteerWheelAngleSign : Inport  Port=2
  canEPS_LKATorqOvrlDlvd : Inport  Port=3
  canEPS_DrvInputTorq : Inport  Port=4
  canSteerWheelSpd : Inport  Port=5
  canSteerWheelSpdSign : Inport  Port=6
  SteerAngleOffset_deg : Inport  Port=7
  eviVxvRef_ms : Inport  Port=8
  desLaneValid : Inport  Port=9
  desLaneA3 : Inport  Port=10
  desLaneA2 : Inport  Port=11
  desLaneA1 : Inport  Port=12
  desLaneA0 : Inport  Port=13
  TarDangerlLevel : Inport  Port=14
  kapTraj : Inport  Port=15
  LaneWidth : Inport  Port=16
  psiDtOpt : Inport  Port=17
  axRef_ms2 : Inport  Port=18
  Constant30 : Constant  Value=0  OutDataTypeStr=single
  Constant31 : Constant  Value=0  OutDataTypeStr=uint8
  Delay : Delay
  Lateral_Control : Subsystem  Variant=on  VariantControlMode=label  LabelModeActiveChoice=kinematics_MPC
  Motion_Planning : Subsystem  Variant=on  VariantControlMode=label  LabelModeActiveChoice=CartesianTrajectoryMPC
  OverRideDetect : Subsystem
  Signal Copy{,1,4,6} (4 alike) : SignalConversion  OverrideOpt=off
  SteerAngleCorrect : Subsystem
  Subsystem : Subsystem
  Terminator{3,5..7,10} (5 alike) : Terminator
  Vehicle_Speed : Subsystem
  TrgSteerAngle : Outport  OutDataTypeStr=single
  epsTrqReqValue : Outport  Port=2
  epsTrqReqFlag : Outport  Port=3
  wires:
  Signal Copy1/1 -> TrgSteerAngle/1  "LCS_LATC_OutTrgSteerAngle"
  Signal Copy/1 -> [LCS_LCC_ref_curve]  "LCS_PLAN_PreviewPointRefCurve"
  [LCS_LCC_ref_theta] -> Lateral_Control/7(Ref_theta)
  Motion_Planning/10(ref_theta) -> [LCS_LCC_ref_theta]  "LCS_PLAN_PreviewPointRefTheta"
  Subsystem/3(DeslaneWidth) -> [DeslaneWidth]
  Subsystem/1(DeslineC0) -> [DeslineC0]
  Subsystem/2(LCS_EqA0) -> [Eq_A0]
  Vehicle_Speed/1(LCS_IN_Spd_Kph) -> [DisplaySpd_kph]
  eviVxvRef_ms/1 -> Vehicle_Speed/1(LCS_IN_Spd_ms), [vRef]
  SteerAngleCorrect/3(SteerAngleSpd_degs) -> [SteerAngleSpd_degs]
  canSteerWheelSpdSign/1 -> SteerAngleCorrect/5(canSteerWheelSpdSign)
  canSteerWheelSpd/1 -> SteerAngleCorrect/4(canSteerWheelSpd)
  OverRideDetect/1(isOverRide) -> [isOvride]
  SteerAngleCorrect/2(LCS_CurSteerAngle_deg) -> [SteerAngle_deg]
  SteerAngleCorrect/1(LCS_IN_CurSteerAngle_deg) -> [LCS_IN_SteerAngle_deg]
  SteerAngleOffset_deg/1 -> SteerAngleCorrect/3(SteerAngleOffset_deg)
  canSteerWheelAngleSign/1 -> SteerAngleCorrect/2(canSteerWheelAngleSign)
  canSteerWheelAngle/1 -> SteerAngleCorrect/1(canSteerWheelAngle)
  [LineValid] -> Motion_Planning/1(DesLineValid)
  [DeslineC0] -> Motion_Planning/2(DesLineC0)
  [SteerAngleOffset_deg] -> Lateral_Control/22(SteerAngleOffset_deg)
  [DeslaneWidth] -> Lateral_Control/21(DesLaneWidth)
  [DeslineC1] -> Lateral_Control/18(DesLineC1)
  [DeslineC2] -> Lateral_Control/19(DesLineC2)
  [DeslineC3] -> Lateral_Control/20(DesLineC3)
  [DeslineC0] -> Lateral_Control/17(DesLineC0)
  Lateral_Control/1(TrgSteerAngle) -> Signal Copy1/1
  [Plan_Trajectory_Theta] -> Lateral_Control/16(Plan_Trajectory_Theta)
  [Plan_Trajectory_Y] -> Lateral_Control/15(Plan_Trajectory_Y)
  [Plan_Trajectory_X] -> Lateral_Control/14(Plan_Trajectory_X)
  [Long_Acc] -> Lateral_Control/13(Long_Acc)
  axRef_ms2/1 -> [Long_Acc]
  [YawRate] -> Lateral_Control/12(YawRate)
  psiDtOpt/1 -> [YawRate]
  [TarDangerLevel] -> Lateral_Control/2(TarDangerLevel)
  [LCS_LCC_heading_error_rate] -> Lateral_Control/11(Heading_error_rate)
  [LCS_LCC_heading_error] -> Lateral_Control/10(Heading_error)
  [LCS_LCC_Later_error_rate] -> Lateral_Control/9(Later_error_rate)
  [LCS_LCC_Later_error] -> Lateral_Control/8(Later_error)
  [LCS_LCC_ref_curve] -> Lateral_Control/6(Ref_curve)
  [LCS_IN_SteerAngle_deg] -> Lateral_Control/5(LCS_SteerAngle_deg)
  [DisplaySpd_kph] -> Lateral_Control/4(Veh_Speed_kph)
  [vRef] -> Lateral_Control/3(Veh_Speed_ms)
  [LineValid] -> Lateral_Control/1(LineValid)
  [kapTraj] -> Motion_Planning/11(kapEgo)
  [TarDangerLevel] -> Motion_Planning/9(TarDangerLevel)
  [DisplaySpd_kph] -> Motion_Planning/8(Veh_Speed_kph)
  [YawRate] -> Motion_Planning/7(YawRate)
  [vRef] -> Motion_Planning/6(Veh_Speed_ms)
  desLaneA3/1 -> Motion_Planning/5(DesLineC3), [DeslineC3]  "LCS_IN_desLaneA3"
  desLaneA2/1 -> [DeslineC2], Motion_Planning/4(DesLineC2)  "LCS_IN_desLaneA2"
  desLaneA1/1 -> [DeslineC1], Motion_Planning/3(DesLineC1)  "LCS_IN_desLaneA1"
  [Long_Acc] -> Motion_Planning/10(Long_Acc)
  Delay/1 -> [TarDangerLevel]  "LCS_IN_TarDangerlLevel_Delay2Frame"
  Motion_Planning/3(PlanTheta) -> [Plan_Trajectory_Theta]  "LCS_PLAN_Trajectory_PlanTheta"
  Motion_Planning/4(idx) -> Terminator7/1  "LCS_PLAN_Trajectory_PlanIdex"
  Motion_Planning/5(PreviewX) -> Terminator6/1  "LCS_PLAN_Trajectory_PreviewX"
  Motion_Planning/6(PreviewY) -> Terminator5/1  "LCS_PLAN_Trajectory_PreviewY"
  Motion_Planning/7(PreviewTheta) -> Terminator3/1  "LCS_PLAN_Trajectory_PreviewTheta"
  [TarDangerlLevel] -> Delay/1
  Constant31/1 -> epsTrqReqFlag/1
  Constant30/1 -> epsTrqReqValue/1
  Motion_Planning/14(heading_error_rate) -> [LCS_LCC_heading_error_rate]  "LCS_PLAN_PreviewPointHeadingErrRate"
  Motion_Planning/13(heading_error) -> [LCS_LCC_heading_error]  "LCS_PLAN_PreviewPointHeadingErr"
  Motion_Planning/12(lateral_error_rate) -> [LCS_LCC_Later_error_rate]  "LCS_PLAN_PreviewPointLaterErrRate"
  Motion_Planning/11(lateral_error) -> [LCS_LCC_Later_error]  "LCS_PLAN_PreviewPointLaterErr"
  Motion_Planning/9(ref_curvature) -> Signal Copy/1
  Motion_Planning/8(numTraj) -> Terminator10/1  "LCS_PLAN_Trajectory_NumTraj"
  Motion_Planning/2(PlanY) -> [Plan_Trajectory_Y]  "LCS_PLAN_Trajectory_PlanY"
  Motion_Planning/1(PlanX) -> [Plan_Trajectory_X]  "LCS_PLAN_TrajectoryX"
  Signal Copy6/1 -> [TarDangerlLevel]  "LCS_IN_TarDangerlLevel"
  Signal Copy4/1 -> [LineValid]  "LCS_IN_desLaneValid"
  desLaneValid/1 -> Signal Copy4/1
  LaneWidth/1 -> Subsystem/2(LaneWidth)
  TarDangerlLevel/1 -> Signal Copy6/1
  kapTraj/1 -> [kapTraj]
  canEPS_LKATorqOvrlDlvd/1 -> [canEPS_LKATorqOvrlDlvd]
  desLaneA0/1 -> Subsystem/1(LCS_IN_desLaneA0)  "LCS_IN_desLaneA0"
  canEPS_DrvInputTorq/1 -> OverRideDetect/1(DrvTrqInput)

== system PvtSubSys_LATC/Subsystem/LateralControl/m//s->kph ==
  m/s : Inport
  Constant5 : Constant  Value=1.3  OutDataTypeStr=single
  Gain3 : Gain  Gain=3.6
  Gain4 : Gain  Gain=1.03
  Sum : Sum  Inputs=|++
  kph : Outport
  wires:
  m/s/1 -> Gain3/1
  Sum/1 -> kph/1
  Gain3/1 -> Gain4/1
  Constant5/1 -> Sum/2
  Gain4/1 -> Sum/1

== system PvtSubSys_LATC/Subsystem/LateralControl/ESS_SteerSpd_Test/LP filter ==
  Raw : Inport
  TorqFilterTime : Inport  Port=2
  Memory2 : Memory  InheritSampleTime=on
  Product1 : Product  RndMeth=Zero
  Product4 : Product  Inputs=*/  RndMeth=Zero
  Sum4 : Sum  Inputs=+-|
  Sum5 : Sum  Inputs=++|
  Weight/N3 : Constant  Value=0.02  OutDataTypeStr=single
  output : Outport
  wires:
  TorqFilterTime/1 -> Product4/2
  Product4/1 -> Product1/1
  Weight/N3/1 -> Product4/1
  Raw/1 -> Sum4/1
  Product1/1 -> Sum5/1
  Sum4/1 -> Product1/2
  Memory2/1 -> Sum4/2, Sum5/2
  Sum5/1 -> Memory2/1, output/1

== system PvtSubSys_LATC/Subsystem/LateralControl/ESS_SteerSpd_Test/LP filter1 ==
  Raw : Inport
  TorqFilterTime : Inport  Port=2
  Memory2 : Memory  InheritSampleTime=on
  Product1 : Product  RndMeth=Zero
  Product4 : Product  Inputs=*/  RndMeth=Zero
  Sum4 : Sum  Inputs=+-|
  Sum5 : Sum  Inputs=++|
  Weight/N3 : Constant  Value=0.02  OutDataTypeStr=single
  output : Outport
  wires:
  Sum5/1 -> output/1, Memory2/1
  Memory2/1 -> Sum5/2, Sum4/2
  Sum4/1 -> Product1/2
  Product1/1 -> Sum5/1
  Raw/1 -> Sum4/1
  Weight/N3/1 -> Product4/1
  Product4/1 -> Product1/1
  TorqFilterTime/1 -> Product4/2

== system PvtSubSys_LATC/Subsystem/LateralControl/ESS_SteerSpd_Test/NotActiveFlgDelayTime ==
  t_offset : Inport
  LCS_ESS_NotActiveFlg : Inport  Port=2
  Constant5 : Constant  Value=0.02  OutDataTypeStr=single
  MATLAB Function : MATLAB Function  TreatAsAtomicUnit=on
  Unit Delay2 : UnitDelay  SampleTime=-1  HasFrameUpgradeWarning=on
  Unit Delay3 : UnitDelay  SampleTime=-1  HasFrameUpgradeWarning=on
  Unit Delay4 : UnitDelay  SampleTime=-1  HasFrameUpgradeWarning=on
  Flg : Outport
  wires:
  MATLAB Function/2(delaytime) -> Unit Delay3/1
  MATLAB Function/3(flg) -> Unit Delay2/1
  LCS_ESS_NotActiveFlg/1 -> MATLAB Function/1(FlgIn)
  Unit Delay2/1 -> MATLAB Function/6(flgK1)
  Constant5/1 -> MATLAB Function/3(tcycle)
  MATLAB Function/1(FlgOut) -> Unit Delay4/1, Flg/1
  t_offset/1 -> MATLAB Function/2(t_offset)
  Unit Delay3/1 -> MATLAB Function/5(delaytimeK1)
  Unit Delay4/1 -> MATLAB Function/4(FlgOutK1)

== system PvtSubSys_LATC/Subsystem/LateralControl/ESS_SteerSpd_Test/Subsystem1 ==
  In1 : Inport
  Add : Sum
  Constant : Constant  Value=Ts
  Constant1 : Constant  Value=0
  Constant2 : Constant  Value=Max
  Max : MinMax  Inputs=2
  Switch : Switch  Criteria=u2 ~= 0
  Unit Delay : UnitDelay  SampleTime=-1  HasFrameUpgradeWarning=on
  Out1 : Outport
  wires:
  Unit Delay/1 -> Add/1
  In1/1 -> Switch/2
  Constant/1 -> Add/2
  Constant1/1 -> Switch/3
  Add/1 -> Switch/1
  Max/1 -> Unit Delay/1, Out1/1
  Constant2/1 -> Max/2
  Switch/1 -> Max/1

== system PvtSubSys_LATC/Subsystem/LateralControl/ESS_SteerSpd_Test/Subsystem10 ==
  In1 : Inport
  Add : Sum
  Constant : Constant  Value=Ts
  Constant1 : Constant  Value=0
  Constant2 : Constant  Value=Max
  Max : MinMax  Inputs=2
  Switch : Switch  Criteria=u2 ~= 0
  Unit Delay : UnitDelay  SampleTime=-1  HasFrameUpgradeWarning=on
  Out1 : Outport
  wires:
  Switch/1 -> Max/1
  Constant2/1 -> Max/2
  Max/1 -> Out1/1, Unit Delay/1
  Add/1 -> Switch/1
  Constant1/1 -> Switch/3
  Constant/1 -> Add/2
  In1/1 -> Switch/2
  Unit Delay/1 -> Add/1

== system PvtSubSys_LATC/Subsystem/LateralControl/ESS_SteerSpd_Test/Subsystem2 ==
  In1 : Inport
  Add : Sum
  Constant : Constant  Value=Ts
  Constant1 : Constant  Value=0
  Constant2 : Constant  Value=Max
  Max : MinMax  Inputs=2
  Switch : Switch  Criteria=u2 ~= 0
  Unit Delay : UnitDelay  SampleTime=-1  HasFrameUpgradeWarning=on
  Out1 : Outport
  wires:
  Unit Delay/1 -> Add/1
  In1/1 -> Switch/2
  Constant/1 -> Add/2
  Constant1/1 -> Switch/3
  Add/1 -> Switch/1
  Max/1 -> Unit Delay/1, Out1/1
  Constant2/1 -> Max/2
  Switch/1 -> Max/1

== system PvtSubSys_LATC/Subsystem/LateralControl/LCS_Angle/Lateral_Control ==
  note: 1) Add Subsystem or Model blocks as valid variant choices.
      | 2) You cannot connect blocks at this level. At simulation, connectivity is automatically
      | determined, based on the active variant and port name matching.
  LineValid : Inport
  TarDangerLevel : Inport  Port=2
  Veh_Speed_ms : Inport  Port=3
  Veh_Speed_kph : Inport  Port=4
  LCS_SteerAngle_deg : Inport  Port=5
  Ref_curve : Inport  Port=6
  Ref_theta : Inport  Port=7
  Later_error : Inport  Port=8
  Later_error_rate : Inport  Port=9
  Heading_error : Inport  Port=10
  Heading_error_rate : Inport  Port=11
  YawRate : Inport  Port=12
  Long_Acc : Inport  Port=13
  Plan_Trajectory_X : Inport  Port=14
  Plan_Trajectory_Y : Inport  Port=15
  Plan_Trajectory_Theta : Inport  Port=16
  DesLineC0 : Inport  Port=17
  DesLineC1 : Inport  Port=18
  DesLineC2 : Inport  Port=19
  DesLineC3 : Inport  Port=20
  DesLaneWidth : Inport  Port=21
  SteerAngleOffset_deg : Inport  Port=22
  Dynamic_Model_LQR : Subsystem  VariantControl=LQR
  MPC : Subsystem  VariantControl=MPC
  kinematics_MPC : Subsystem  VariantControl=kinematics_MPC
  TrgSteerAngle : Outport  OutDataTypeStr=single

== system PvtSubSys_LATC/Subsystem/LateralControl/LCS_Angle/Motion_Planning ==
  note: 1) Add Subsystem or Model blocks as valid variant choices.
      | 2) You cannot connect blocks at this level. At simulation, connectivity is automatically
      | determined, based on the active variant and port name matching.
  DesLineValid : Inport
  DesLineC0 : Inport  Port=2
  DesLineC1 : Inport  Port=3
  DesLineC2 : Inport  Port=4
  DesLineC3 : Inport  Port=5
  Veh_Speed_ms : Inport  Port=6
  YawRate : Inport  Port=7
  Veh_Speed_kph : Inport  Port=8
  TarDangerLevel : Inport  Port=9
  Long_Acc : Inport  Port=10
  kapEgo : Inport  Port=11
  CartesianTrajectory : Subsystem  VariantControl=CartesianTrajectory
  CartesianTrajectory_MPC : Subsystem  VariantControl=CartesianTrajectoryMPC
  FrenetTrajectory : Subsystem  VariantControl=FrenetTrajectory
  FrenetTrajectory_Lateral : Subsystem  VariantControl=FrenetTrajectory_Lateral
  PlanX : Outport
  PlanY : Outport  Port=2
  PlanTheta : Outport  Port=3
  idx : Outport  Port=4
  PreviewX : Outport  Port=5
  PreviewY : Outport  Port=6
  PreviewTheta : Outport  Port=7
  numTraj : Outport  Port=8
  ref_curvature : Outport  Port=9
  ref_theta : Outport  Port=10
  lateral_error : Outport  Port=11
  lateral_error_rate : Outport  Port=12
  heading_error : Outport  Port=13
  heading_error_rate : Outport  Port=14

== system PvtSubSys_LATC/Subsystem/LateralControl/LCS_Angle/OverRideDetect ==
  DrvTrqInput : Inport
  Abs4 : Abs
  Chart : Stateflow chart  TreatAsAtomicUnit=on
  Compare To Constant1 : simulink/Logic and Bit Operations/Compare To Constant  relop=>  const=P_LCS_OverRideTime_TH_s  OutDataTypeStr=boolean
  Compare To Constant2 : simulink/Logic and Bit Operations/Compare To Constant  relop=>  const=P_LCS_NoOverRideTime_TH_s  OutDataTypeStr=boolean
  Compare To Constant3 : simulink/Logic and Bit Operations/Compare To Constant  relop=>  const=P_LCS_DetOverRide_DrvTrq_TH  OutDataTypeStr=boolean
  Compare To Constant4 : simulink/Logic and Bit Operations/Compare To Constant  relop=<=  const=P_LCS_DetNoOverRide_DrvTrq_TH  OutDataTypeStr=boolean
  Constant12 : Constant  Value=0.8
  Constant13 : Constant  Value=true
  Constant15 : Constant  Value=P_LCS_OverRideDetect_b
  LP filter4 : Subsystem
  Logical Operator1 : Logic  AllPortsSameDT=off  OutDataTypeStr=boolean
  Subsystem17 : Subsystem  mask{Ts=0.02, Max=10}
      mask prompts: Ts "Sample Time:"; Max "Max Limit:"
      mask Display:
      | Ts=get_param(gcb,'Ts');
      | Max=get_param(gcb,'Max');
      | disp(['Ts:' Ts '\n' 'Max:' Max ]);
  Subsystem4 : Subsystem  mask{Ts=0.02, Max=10}
      mask prompts: Ts "Sample Time:"; Max "Max Limit:"
      mask Display:
      | Ts=get_param(gcb,'Ts');
      | Max=get_param(gcb,'Max');
      | disp(['Ts:' Ts '\n' 'Max:' Max ]);
  isOverRide : Outport
  wires:
  Constant15/1 -> Logical Operator1/1
  Logical Operator1/1 -> isOverRide/1
  Chart/1(isOverRide) -> Logical Operator1/2  "LCS_OverRideDetect_b"
  Compare To Constant2/1 -> Chart/2(NoOvride)
  Compare To Constant1/1 -> Chart/1(Ovride)
  DrvTrqInput/1 -> Abs4/1
  Constant13/1 -> LP filter4/3(enable)
  Compare To Constant3/1 -> Subsystem4/1(In1)
  LP filter4/1(output) -> Compare To Constant3/1, Compare To Constant4/1
  Constant12/1 -> LP filter4/2(TorqFilterTime)
  Abs4/1 -> LP filter4/1(Raw)
  Subsystem4/1(Out1) -> Compare To Constant1/1
  Subsystem17/1(Out1) -> Compare To Constant2/1
  Compare To Constant4/1 -> Subsystem17/1(In1)

== system PvtSubSys_LATC/Subsystem/LateralControl/LCS_Angle/SteerAngleCorrect ==
  canSteerWheelAngle : Inport
  canSteerWheelAngleSign : Inport  Port=2
  SteerAngleOffset_deg : Inport  Port=3
  canSteerWheelSpd : Inport  Port=4
  canSteerWheelSpdSign : Inport  Port=5
  Add1 : Sum  Inputs=+-
  Bias1 : Bias  Bias=-0.5
  Bias2 : Bias  Bias=-0.5
  Gain2 : Gain  Gain=-2
  Gain5 : Gain  Gain=-2
  Product4 : Product
  Product5 : Product
  LCS_IN_CurSteerAngle_deg : Outport
  LCS_CurSteerAngle_deg : Outport  Port=2
  SteerAngleSpd_degs : Outport  Port=3
  wires:
  Bias2/1 -> Gain2/1
  canSteerWheelSpdSign/1 -> Bias2/1
  canSteerWheelSpd/1 -> Product4/1
  Product4/1 -> SteerAngleSpd_degs/1  "LCS_IN_SteerAngleSpd_degs"
  Gain2/1 -> Product4/2
  canSteerWheelAngle/1 -> Product5/1
  Add1/1 -> LCS_CurSteerAngle_deg/1  "LCS_CurSteerAngle_deg"
  canSteerWheelAngleSign/1 -> Bias1/1
  Gain5/1 -> Product5/2
  Bias1/1 -> Gain5/1
  Product5/1 -> Add1/1, LCS_IN_CurSteerAngle_deg/1  "LCS_IN_CurSteerAngle_deg"
  SteerAngleOffset_deg/1 -> [SteerAngleOffset_deg], Add1/2

== system PvtSubSys_LATC/Subsystem/LateralControl/LCS_Angle/Subsystem ==
  LCS_IN_desLaneA0 : Inport
  LaneWidth : Inport  Port=2
  Abs1 : Abs
  Constant4 : Constant  Value=3.6  OutDataTypeStr=single
  Constant6 : Constant  Value=3  OutDataTypeStr=single
  Constant7 : Constant  Value=4  OutDataTypeStr=single
  Divide : Product  Inputs=**/
  MinMax : MinMax  Function=max  Inputs=2
  MinMax1 : MinMax  Inputs=2
  DeslineC0 : Outport
  LCS_EqA0 : Outport  Port=2
  DeslaneWidth : Outport  Port=3
  wires:
  LCS_IN_desLaneA0/1 -> Abs1/1, DeslineC0/1
  Constant7/1 -> MinMax1/2
  Divide/1 -> LCS_EqA0/1  "LCS_EqA0"
  LaneWidth/1 -> MinMax/1, DeslaneWidth/1
  Abs1/1 -> Divide/1
  Constant4/1 -> Divide/3
  Constant6/1 -> MinMax/2
  MinMax/1 -> MinMax1/1
  MinMax1/1 -> Divide/2

== system PvtSubSys_LATC/Subsystem/LateralControl/LCS_Angle/Vehicle_Speed ==
  LCS_IN_Spd_ms : Inport
  Constant8 : Constant  Value=1.3  OutDataTypeStr=single
  Gain3 : Gain  Gain=3.6
  Gain4 : Gain  Gain=1.03
  Sum : Sum  Inputs=|++
  LCS_IN_Spd_Kph : Outport
  wires:
  Gain4/1 -> Sum/1
  Sum/1 -> LCS_IN_Spd_Kph/1  "LCS_IN_Spd_Kph"
  Constant8/1 -> Sum/2
  LCS_IN_Spd_ms/1 -> Gain3/1
  Gain3/1 -> Gain4/1

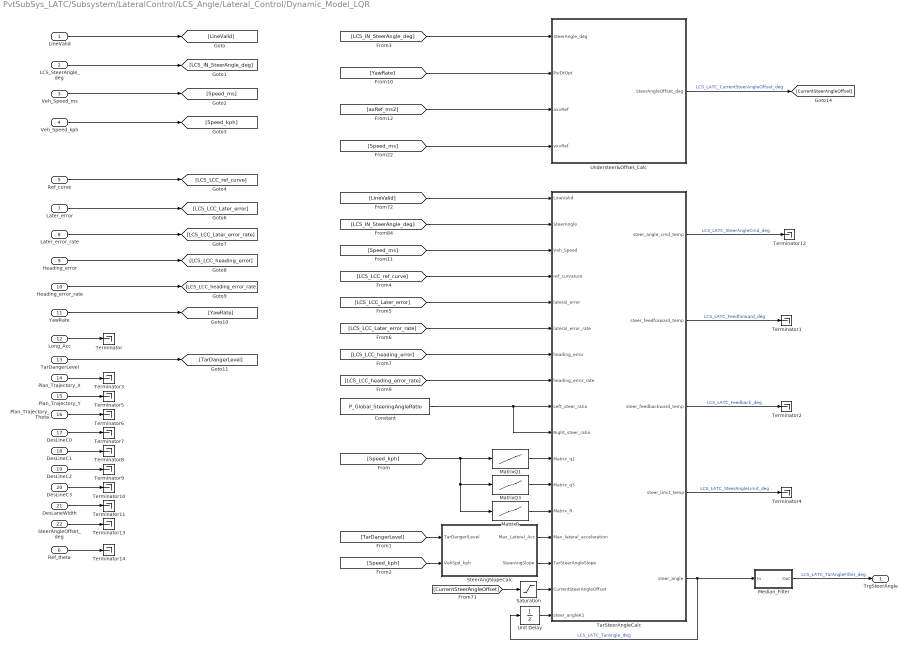
== system PvtSubSys_LATC/Subsystem/LateralControl/LCS_Angle/Lateral_Control/Dynamic_Model_LQR ==
  LineValid : Inport
  LCS_SteerAngle_deg : Inport  Port=2
  Veh_Speed_ms : Inport  Port=3
  Veh_Speed_kph : Inport  Port=4
  Ref_curve : Inport  Port=5
  Ref_theta : Inport  Port=6
  Later_error : Inport  Port=7
  Later_error_rate : Inport  Port=8
  Heading_error : Inport  Port=9
  Heading_error_rate : Inport  Port=10
  YawRate : Inport  Port=11
  Long_Acc : Inport  Port=12
  TarDangerLevel : Inport  Port=13
  Plan_Trajectory_X : Inport  Port=14
  Plan_Trajectory_Y : Inport  Port=15
  Plan_Trajectory_Theta : Inport  Port=16
  DesLineC0 : Inport  Port=17
  DesLineC1 : Inport  Port=18
  DesLineC2 : Inport  Port=19
  DesLineC3 : Inport  Port=20
  DesLaneWidth : Inport  Port=21
  SteerAngleOffset_deg : Inport  Port=22
  Constant : Constant  Value=P_Global_SteeringAngleRatio  OutDataTypeStr=single
  MatrixQ1 : Lookup_n-D  NumberOfTableDimensions=1  BreakpointsForDimension1=P_LCS_VehicleSpd_TabX_Kph  Table=P_LCS_LATC_MatrixQ1_st  ExtrapMethod=Clip  UseLastTableValue=on  InternalRulePriority=Speed  RndMeth=Simplest  InputSameDT=on
  MatrixQ3 : Lookup_n-D  NumberOfTableDimensions=1  BreakpointsForDimension1=P_LCS_VehicleSpd_TabX_Kph  Table=P_LCS_LATC_MatrixQ3_st  ExtrapMethod=Clip  UseLastTableValue=on  InternalRulePriority=Speed  RndMeth=Simplest  InputSameDT=on
  MatrixR : Lookup_n-D  NumberOfTableDimensions=1  BreakpointsForDimension1=P_LCS_VehicleSpd_TabX_Kph  Table=P_LCS_LATC_MatrixR_st  ExtrapMethod=Clip  UseLastTableValue=on  InternalRulePriority=Speed  RndMeth=Simplest  InputSameDT=on
  Median_Filter : Subsystem
  Saturation : Saturate  UpperLimit=8  LowerLimit=-8  OutDataTypeStr=single
  SteerAngSlopeCalc : Subsystem
  TarSteerAngleCalc : MATLAB Function  TreatAsAtomicUnit=on
  Terminator{,1..14} (15 alike) : Terminator
  Understeer&Offset_Calc : Subsystem
  Unit Delay : UnitDelay  SampleTime=-1  HasFrameUpgradeWarning=on
  TrgSteerAngle : Outport  OutDataTypeStr=single
  wires:
  Ref_theta/1 -> Terminator14/1
  MatrixR/1 -> TarSteerAngleCalc/13(Matrix_R)
  SteerAngleOffset_deg/1 -> Terminator13/1
  DesLaneWidth/1 -> Terminator11/1
  DesLineC3/1 -> Terminator10/1
  DesLineC2/1 -> Terminator9/1
  DesLineC1/1 -> Terminator8/1
  DesLineC0/1 -> Terminator7/1
  Plan_Trajectory_Theta/1 -> Terminator6/1
  Plan_Trajectory_Y/1 -> Terminator5/1
  Plan_Trajectory_X/1 -> Terminator3/1
  Long_Acc/1 -> Terminator/1
  TarDangerLevel/1 -> [TarDangerLevel]
  YawRate/1 -> [YawRate]
  Heading_error_rate/1 -> [LCS_LCC_heading_error_rate]
  Heading_error/1 -> [LCS_LCC_heading_error]
  Later_error_rate/1 -> [LCS_LCC_Later_error_rate]
  Later_error/1 -> [LCS_LCC_Later_error]
  Ref_curve/1 -> [LCS_LCC_ref_curve]
  Veh_Speed_kph/1 -> [Speed_kph]
  Veh_Speed_ms/1 -> [Speed_ms]
  LCS_SteerAngle_deg/1 -> [LCS_IN_SteerAngle_deg]
  LineValid/1 -> [LineValid]
  [LCS_IN_SteerAngle_deg] -> Understeer&Offset_Calc/1(SteerAngle_deg)
  [axRef_ms2] -> Understeer&Offset_Calc/3(axvRef)
  Understeer&Offset_Calc/1(SteerAngleOffset_deg) -> [CurrentSteerAngleOffset]  "LCS_LATC_CurrentSteerAngleOffset_deg"
  [YawRate] -> Understeer&Offset_Calc/2(PsiDtOpt)
  [Speed_ms] -> Understeer&Offset_Calc/4(vxvRef)
  MatrixQ1/1 -> TarSteerAngleCalc/11(Matrix_q1)
  MatrixQ3/1 -> TarSteerAngleCalc/12(Matrix_q3)
  [Speed_ms] -> TarSteerAngleCalc/3(Veh_Speed)
  SteerAngSlopeCalc/2(SteerAngSlope) -> TarSteerAngleCalc/15(TarSteerAngleSlope)
  Median_Filter/1(Out) -> TrgSteerAngle/1  "LCS_LATC_TarAngleFilter_deg"
  [CurrentSteerAngleOffset] -> Saturation/1
  SteerAngSlopeCalc/1(Max_Lateral_Acc) -> TarSteerAngleCalc/14(Max_lateral_acceleration)
  [LCS_LCC_ref_curve] -> TarSteerAngleCalc/4(ref_curvature)
  [LCS_LCC_heading_error_rate] -> TarSteerAngleCalc/8(heading_error_rate)
  [LCS_LCC_Later_error_rate] -> TarSteerAngleCalc/6(lateral_error_rate)
  [LCS_LCC_heading_error] -> TarSteerAngleCalc/7(heading_error)
  [TarDangerLevel] -> SteerAngSlopeCalc/1(TarDangerlLevel)
  [LCS_LCC_Later_error] -> TarSteerAngleCalc/5(lateral_error)
  Saturation/1 -> TarSteerAngleCalc/16(CurrentSteerAngleOffset)
  TarSteerAngleCalc/1(steer_angle_cmd_temp) -> Terminator12/1  "LCS_LATC_SteerAngleCmd_deg"
  [LineValid] -> TarSteerAngleCalc/1(LineValid)
  [Speed_kph] -> MatrixR/1, MatrixQ3/1, MatrixQ1/1
  Unit Delay/1 -> TarSteerAngleCalc/17(steer_angleK1)
  TarSteerAngleCalc/4(steer_limit_temp) -> Terminator4/1  "LCS_LATC_SteerAngleLimit_deg"
  [Speed_kph] -> SteerAngSlopeCalc/2(VehSpd_kph)
  Constant/1 -> TarSteerAngleCalc/9(Left_steer_ratio), TarSteerAngleCalc/10(Right_steer_ratio)
  TarSteerAngleCalc/2(steer_feedforward_temp) -> Terminator1/1  "LCS_LATC_Feedforward_deg"
  TarSteerAngleCalc/5(steer_angle) -> Unit Delay/1, Median_Filter/1(In)  "LCS_LATC_TarAngle_deg"
  TarSteerAngleCalc/3(steer_feedbackward_temp) -> Terminator2/1  "LCS_LATC_Feedback_deg"
  [LCS_IN_SteerAngle_deg] -> TarSteerAngleCalc/2(SteerAngle)
